simulink model "getWheelAngle"  (R2019a)
settings: Solver=FixedStepAuto  StartTime=0.0  StopTime=inf  FixedStep=Ts  RelTol=1e-3  EnableMultiTasking=on
libraries: dspstat3 x2
settings Model: SimulationMode=external  Creator=bspoe  LastModifiedBy=florian
settings SolverCC: PositivePriorityOrder=on
settings OptimizationCC: EnhancedBackFolding=on  PassReuseOutputArgsAs=Individual arguments  MaxStackSize=64  OptimizeBlockOrder=speed  DifferentSizesBufferReuse=on  OptimizationCustomize=off
settings DebuggingCC: ParameterTunabilityLossMsg=error
settings HardwareCC: ProdBitPerPointer=32  ProdBitPerSizeT=32  ProdBitPerPtrDiffT=32  ProdLargestAtomicInteger=Long  ProdLargestAtomicFloat=Double  ProdWordSize=32  ProdLongLongMode=on  ProdHWDeviceType=ARM Compatible->ARM Cortex
settings SFSimCC: MATLABDynamicMemAlloc=off
settings RTWCC: SystemTargetFile=ert.tlc  HardwareBoard=Raspberry Pi  TLCOptions="-aInlineSetEventsForThisBaseRateFcn=TLC_FALSE -aSuppressMultiTaskScheduler=TLC_FALSE  -aRateBasedStepFcn=0"  TemplateMakefile=ert_default_tmf  GenerateReport=on  Toolchain=GNU GCC Raspberry Pi  IncludeHyperlinkInReport=on  LaunchReport=on  GenerateTraceInfo=on  GenerateTraceReport=on  GenerateTraceReportSl=on  GenerateTraceReportSf=on  GenerateTraceReportEml=on
settings CodeAppCC: ForceParamTrailComments=on  IgnoreCustomStorageClasses=off  OperatorAnnotations=on  SimulinkDataObjDesc=on  SFDataObjDesc=on  InsertBlockDesc=on
settings ERTTargetCC: SupportVariableSizeSignals=on

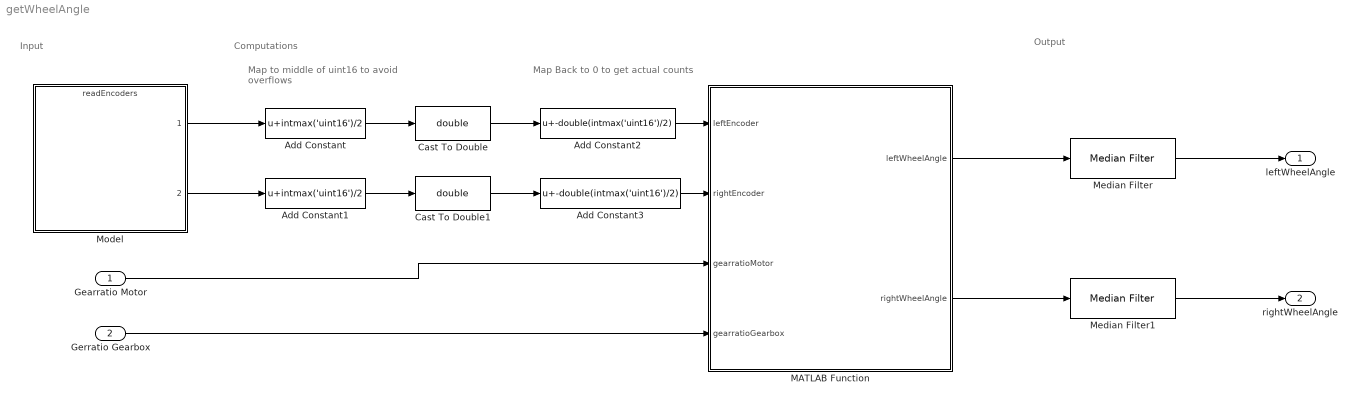
== system getWheelAngle ==
  note: Map to middle of uint16
      | to avoid overflows
  note: Output
  note: Input
  note: Computations
  note: Map Back to 0 to get
      | actual counts
  Gearratio Motor : Inport
  Gerratio Gearbox : Inport  Port=2
  Add Constant : Bias  Bias=intmax('uint16')/2
  Add Constant1 : Bias  Bias=intmax('uint16')/2
  Add Constant2 : Bias  Bias=-double(intmax('uint16')/2)
  Add Constant3 : Bias  Bias=-double(intmax('uint16')/2)
  Cast To Double : DataTypeConversion  OutDataTypeStr=double
  Cast To Double1 : DataTypeConversion  OutDataTypeStr=double
  MATLAB Function : MATLAB Function  TreatAsAtomicUnit=on
  Median Filter : dspstat3/Median Filter  WindowLength=5  SimulateUsing=Interpreted execution
      settings: SourceProductName=DSP System Toolbox  SourceProductBaseCode=DS
  Median Filter1 : dspstat3/Median Filter  WindowLength=5  SimulateUsing=Interpreted execution
      settings: SourceProductName=DSP System Toolbox  SourceProductBaseCode=DS
  Model : ModelReference  ModelNameDialog=readEncoders.slx  SimulationMode=Normal  ModelReferenceVersion=1.9
  leftWheelAngle : Outport
  rightWheelAngle : Outport  Port=2
  wires:
  Model/1 -> Add Constant/1
  Model/2 -> Add Constant1/1
  MATLAB Function/1(leftWheelAngle) -> Median Filter/1
  MATLAB Function/2(rightWheelAngle) -> Median Filter1/1
  Add Constant/1 -> Cast To Double/1
  Add Constant1/1 -> Cast To Double1/1
  Cast To Double/1 -> Add Constant2/1
  Cast To Double1/1 -> Add Constant3/1
  Add Constant3/1 -> MATLAB Function/2(rightEncoder)
  Add Constant2/1 -> MATLAB Function/1(leftEncoder)
  Gerratio Gearbox/1 -> MATLAB Function/4(gearratioGearbox)
  Gearratio Motor/1 -> MATLAB Function/3(gearratioMotor)
  Median Filter/1 -> leftWheelAngle/1
  Median Filter1/1 -> rightWheelAngle/1

== matlab function getWheelAngle/MATLAB Function ==
  data: leftEncoder input; leftWheelAngle output; rightEncoder input; rightWheelAngle output; gearratioMotor input; gearratioGearbox input
function [leftWheelAngle, rightWheelAngle] = calculateWheelAngle(leftEncoder, rightEncoder, gearratioMotor, gearratioGearbox)
%Divide the ticks by the absolute number of ticks per rotation
%and multiply by 2pi
leftWheelAngle = leftEncoder * 2 * pi / (12 * gearratioMotor * gearratioGearbox);

rightWheelAngle = rightEncoder * 2 * pi / (12 * gearratioMotor * gearratioGearbox);
